simulink model "Sys_OL"  (R2025b)
settings: Solver=VariableStepAuto  StartTime=0.0  StopTime=500  RelTol=1e-3
values from neighbouring files (symbols this model uses):
  C = [1, 0, 0]    [fase1.m]
undefined symbols (not defined in the file or in its folder): ueq
settings Model: Creator=Rika  LastModifiedBy=Rika

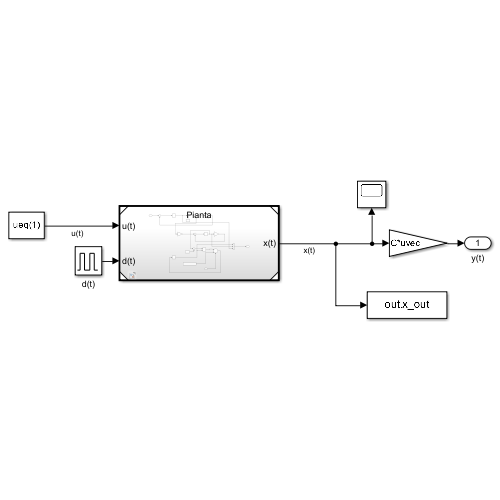
[thumbnail: Simulink's stored preview of the top-level diagram]
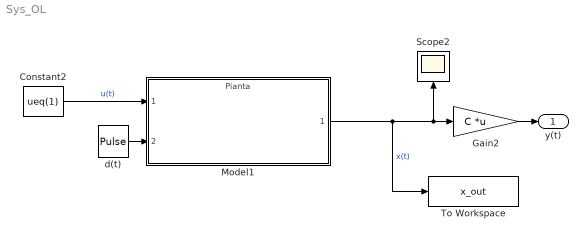
== system Sys_OL ==
  Constant2 : Constant  Value=ueq(1)
  Gain2 : Gain  Gain=C  Multiplication=Matrix(K*u) (u vector)
  Model1 : ModelReference  ModelNameDialog=Pianta.slx  SimulationMode=Normal  ModelReferenceVersion=1.15
  Scope2 : Scope
      settings: ActiveDisplayYMinimum=-163.64284289278072  ActiveDisplayYMaximum=557.05101768268139  DataLoggingVariableName=ScopeData2
  To Workspace : ToWorkspace  VariableName=x_out  SampleTime=-1
  d(t) : DiscretePulseGenerator  PulseType=Time based  Amplitude=10  Period=1000  PulseWidth=3  PhaseDelay=10
  y(t) : Outport
  wires:
  Gain2/1 -> y(t)/1
  Model1/1 -> To Workspace/1, Scope2/1, Gain2/1  "x(t)"
  Constant2/1 -> Model1/1  "u(t)"
  d(t)/1 -> Model1/2
